simulink model "example"  (R2024b)
settings: Solver=VariableStepAuto  StartTime=0.0  StopTime=10.0  RelTol=1e-3
settings Model: Creator=Arhaan  LastModifiedBy=Arhaan

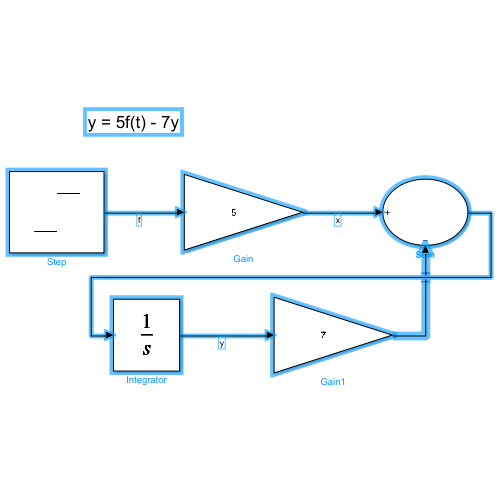
[thumbnail: Simulink's stored preview of the top-level diagram]
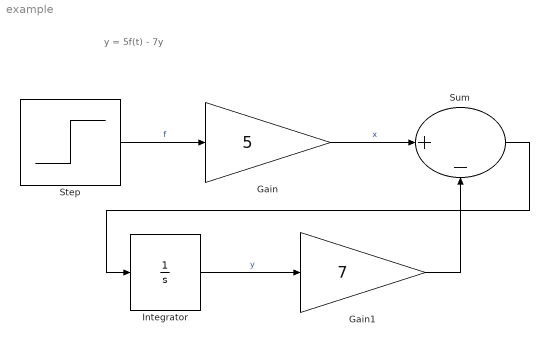
== system example ==
  note: y = 5f(t) - 7y
  Gain : Gain  Gain=5
  Gain1 : Gain  Gain=7
  Integrator : Integrator
  Step : Step  SampleTime=0
  Sum : Sum  Inputs=|+-
  wires:
  Step/1 -> Gain/1  "f"
  Gain/1 -> Sum/1  "x"
  Gain1/1 -> Sum/2
  Integrator/1 -> Gain1/1  "y"
  Sum/1 -> Integrator/1
